simulink model "lab2_schema_sarcina5"  (R2023b)
settings: Solver=ode45  StartTime=0.0  StopTime=200  RelTol=1e-3
settings Model: Creator=Daniela  LastModifiedBy=Daniela

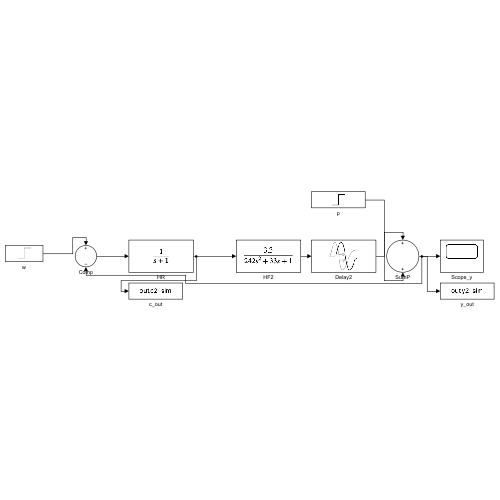
[thumbnail: Simulink's stored preview of the top-level diagram]
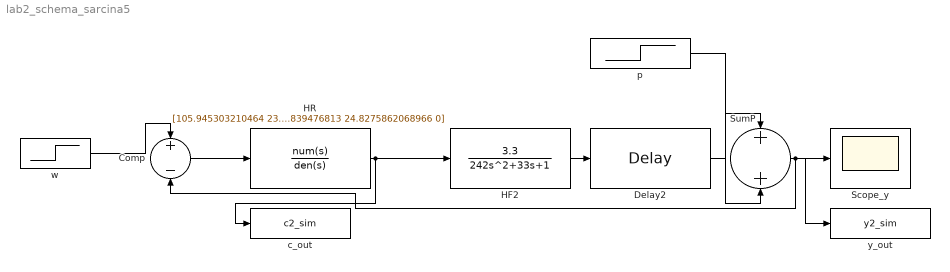
== system lab2_schema_sarcina5 ==
  Comp : Sum  Inputs=+-
  Delay2 : TransportDelay  DelayTime=5
  HF2 : TransferFcn  Numerator=3.3  Denominator=[242 33 1]
  HR : TransferFcn  Numerator=[105.945303210464 23.6637931034483 0.9375]  Denominator=[10.2734839476813 24.8275862068966 0]
  Scope_y : Scope
  SumP : Sum
  c_out : ToWorkspace  VariableName=c2_sim  SampleTime=-1
  p : Step  Time=0  After=0  SampleTime=0
  w : Step  Time=0  SampleTime=0
  y_out : ToWorkspace  VariableName=y2_sim  SampleTime=-1
  wires:
  w/1 -> Comp/1
  Comp/1 -> HR/1
  HR/1 -> HF2/1, c_out/1
  HF2/1 -> Delay2/1
  Delay2/1 -> SumP/1
  p/1 -> SumP/2
  SumP/1 -> Scope_y/1, y_out/1, Comp/2
